simulink model "bit_simulink"  (R2023b)
settings: Solver=FixedStepAuto  StartTime=0.0  StopTime=1000  FixedStep=0.001  MaxStep=0.005  RelTol=1e-3
values from neighbouring files (symbols this model uses):
  d_theta_dt_0 = [0.,0.,0.,0.,0.,0.,0.,0.,0.]'    [Initialization.m]    (also in init_func.m; init_func_env_test.m; main_func.m; sim_loop_rust.m = double([0.,0.,0.,0.,0.,0.,0.,0.,0.]'))
  theta_0 = [0.,0.4*pi/180.0,0.4*pi/180.0,0.1*pi/180.0,0.1*pi/180.0,0.1*pi/180.0,0.,0.1,40*pi/180]'    [Initialization.m]    (also in init_func.m = [0,0,0,0,0,0,0,0,0,0]'; init_func_env_test.m = [0,0,0,0,0,0,0,0,0,0]'; main_func.m = [0.,0.4*pi/180.0,0.4*pi/180.0,0.1*pi/180.0,0.1*pi/180.0,0.1*; sim_loop_rust.m = 0*[0,0,0,0,0,0.0,0,0,-40*pi/180]')
  x0 = [d_theta_dt_0; theta_0; hs_rw]    [main.m]    (also in main_func.m; opt_ql.m = ones(91,1); sim_loop_rust.m = x0*1.01; sim_loop_wind.m)
undefined symbols (not defined in the file or in its folder): Klqr, Klqr_p, Klqr_r, ns, p, Qcm, r_pit, r_roll, rstr, sstr
settings Model: Creator=bholder  LastModifiedBy=bholder

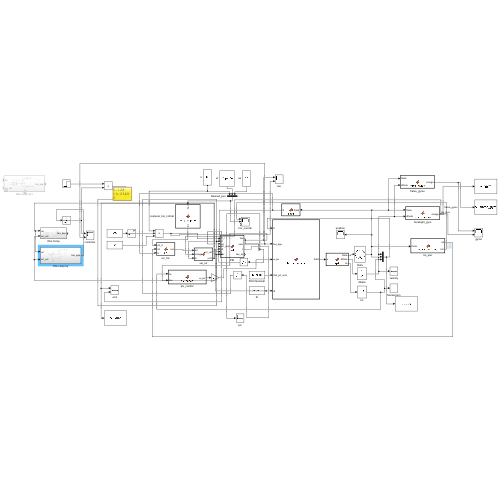
[thumbnail: Simulink's stored preview of the top-level diagram]
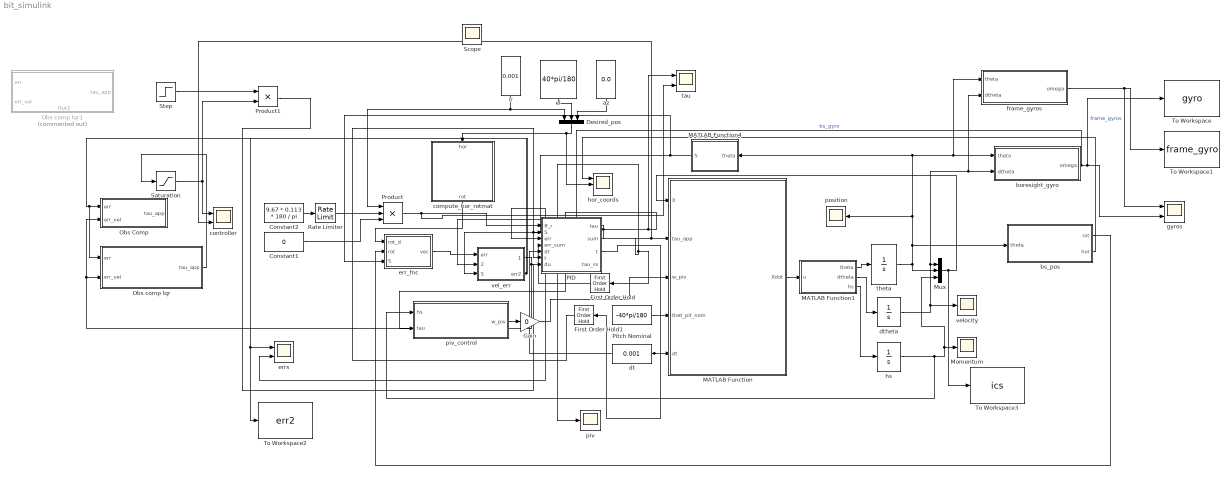
== system bit_simulink ==
  Constant1 : Constant  Value=0
  Constant2 : Constant  Value=9.67 * 0.113 * 180 / pi
  Desired_pos : Mux  Inputs=3
  First Order Hold : FirstOrderHold  InitialOutput=zeros(3,1)  ErrorTolerance=10  AllowContinuousInput=on
  First Order Hold1 : FirstOrderHold  ErrorTolerance=10  AllowContinuousInput=on
  Gain : Gain  Gain=0
  MATLAB Function : MATLAB Function  TreatAsAtomicUnit=on
  MATLAB Function1 : MATLAB Function  TreatAsAtomicUnit=on
  MATLAB Function4 : MATLAB Function  TreatAsAtomicUnit=on
  Momentum : Scope
  Mux : Mux  Inputs=3
  Obs Comp : Subsystem
  Obs comp lqr : Subsystem
  Obs comp lqr1 : Subsystem  Commented=on
      settings: PortSchema="{\"entries\":[{\"content\":{\"sides\":[{\"content\":{\"connectorIds\":[\"In1\",\"In2\"]},\"type\":\"ConnectorPlacement.EquallySpacedRectSide\",\"uuid\":\"f9d8c282-cd97-41f4-aac3-c7cf1abd67fe\"},{\"content\":{\"connectorIds\":[\"Out1\"],\"side\":\"RIGHT\"},\"type\":\"ConnectorPlacement.EquallySpacedRectSide\",\"uuid\":\"09112819-b147-4feb-a738-ff15dc4c45ff\"},{\"content\":{\"side\":\"TOP\"},\"type\":\"ConnectorPlacement.EquallySpacedRectSide\",\"uuid\":\"cd0336e0-d679-46ce-94e8-540b25d3be2c\"},{\"content\":{\"connectorIds\":[\"Out2\"],\"side\":\"BOTTOM\"},\"type\":\"ConnectorPlacement.EquallySpacedRectSide\",\"uuid\":\"8134ff57-d3b4-4301-9a67-166d46c0ba79\"}]},\"type\":\"ConnectorPlacement.EquallySpacedConnector\",\"uuid\":\"7e617e88-15c2-4d81-bfcb-fc8957304092\"}],\"packageUris\":[\"http://schema.mathworks.com/mf0/Connector/R2020b\"],\"version\":\"1.0\"}"
  PID : MATLAB Function  TreatAsAtomicUnit=on
  Pitch Nominal : Constant  Value=-40*pi/180
  Product : Product  Inputs=3
  Product1 : Product
  Rate Limiter : RateLimiter  RisingSlewLimit=15  FallingSlewLimit=-0.25  SampleTimeMode=inherited
  Saturation : Saturate  UpperLimit=1  LowerLimit=-1
  Step : Step  Time=0  Before=1  SampleTime=0
  To Workspace : ToWorkspace  VariableName=gyro  SaveFormat=Timeseries  SampleTime=-1
  To Workspace1 : ToWorkspace  VariableName=frame_gyro  SaveFormat=Timeseries  SampleTime=-1
  To Workspace2 : ToWorkspace  VariableName=err2  SaveFormat=Timeseries  SampleTime=-1
  To Workspace3 : ToWorkspace  VariableName=ics  SaveFormat=Timeseries  SampleTime=-1
      settings: MaxDataPoints=1
  az : Constant  Value=0.0
  boresight_gyro : MATLAB Function  TreatAsAtomicUnit=on
  bs_pos : MATLAB Function  TreatAsAtomicUnit=on
  compute_hor_rotmat : MATLAB Function  TreatAsAtomicUnit=on
  controller : Scope  NumInputPorts=2
  dt : Constant  Value=0.001
  dtheta : Integrator  InitialCondition=d_theta_dt_0  ContinuousStateAttributes='dtheta'
  el : Constant  Value=40*pi/180
  err_fnc : MATLAB Function  TreatAsAtomicUnit=on
  errs : Scope  NumInputPorts=2
  frame_gyros : MATLAB Function  TreatAsAtomicUnit=on
  gyros : Scope  NumInputPorts=2
  hor_coords : Scope  NumInputPorts=3
  hs : Integrator  InitialCondition=x0(19:21)  LimitOutput=on  UpperSaturationLimit=4*pi*4.5  LowerSaturationLimit=-4*pi*4.5  ContinuousStateAttributes='hs'
  ir : Constant  Value=0.001
  piv : Scope
  piv_control : MATLAB Function  TreatAsAtomicUnit=on
  position : Scope
  tau : Scope  NumInputPorts=2
  theta : Integrator  InitialCondition=theta_0  UpperSaturationLimit=1  LowerSaturationLimit=0  WrapState=on  ContinuousStateAttributes='theta'
  vel_err : MATLAB Function  TreatAsAtomicUnit=on
  velocity : Scope
  Scope : Scope
  wires:
  MATLAB Function/1(Xdot) -> MATLAB Function1/1(u)
  MATLAB Function1/2(dtheta) -> dtheta/1
  MATLAB Function1/1(theta) -> theta/1
  theta/1 -> Mux/2, bs_pos/1(theta), MATLAB Function4/1(theta), frame_gyros/1(theta), boresight_gyro/1(theta), position/1
  dtheta/1 -> frame_gyros/2(dtheta), boresight_gyro/2(dtheta), Mux/1, velocity/1
  Mux/1 -> MATLAB Function/1(X), To Workspace3/1
  Pitch Nominal/1 -> MATLAB Function/4(thet_pit_nom)
  dt/1 -> MATLAB Function/5(dt), PID/5(dt)
  MATLAB Function1/3(hs) -> hs/1
  hs/1 -> piv_control/1(hs), Momentum/1, Mux/3
  ir/1 -> Product/1, Desired_pos/1
  Desired_pos/1 -> compute_hor_rotmat/1(hor), hor_coords/2
  az/1 -> Desired_pos/3
  el/1 -> Desired_pos/2
  compute_hor_rotmat/1(rot) -> err_fnc/1(rot_d)
  bs_pos/1(rot) -> err_fnc/2(rot)
  err_fnc/1(vec) -> vel_err/1(err)
  MATLAB Function4/1(S) -> err_fnc/3(S), vel_err/3(S), PID/2(S)
  PID/2(sum) -> piv/1, First Order Hold/1
  First Order Hold/1 -> PID/4(err_sum)
  Constant2/1 -> Rate Limiter/1
  PID/1(tau) -> controller/2, MATLAB Function/2(tau_app), piv_control/2(tau), tau/1
  Rate Limiter/1 -> Product/2
  Constant1/1 -> Product/3
  Product/1 -> tau/2, PID/1(ff_r)
  piv_control/1(w_piv) -> Gain/1
  Gain/1 -> MATLAB Function/3(w_piv)
  PID/3(t) -> First Order Hold1/1
  First Order Hold1/1 -> PID/6("t ")
  boresight_gyro/1(omega) -> To Workspace/1, gyros/2, vel_err/2(omega)  "bs_gyro"
  bs_pos/2(hor) -> hor_coords/1
  frame_gyros/1(omega) -> gyros/1, To Workspace1/1  "frame_gyros"
  vel_err/1(err_vel) -> Obs Comp/2(err_vel), Obs comp lqr/2(err_vel), PID/3(err), errs/2
  vel_err/2(err2) -> To Workspace2/1, errs/1, Obs comp lqr/1(err), Obs Comp/1(err)
  Saturation/1 -> controller/1, Product1/2
  Product1/1 -> PID/7(du)
  Step/1 -> Product1/1
  Obs comp lqr/1(tau_app) -> Saturation/1

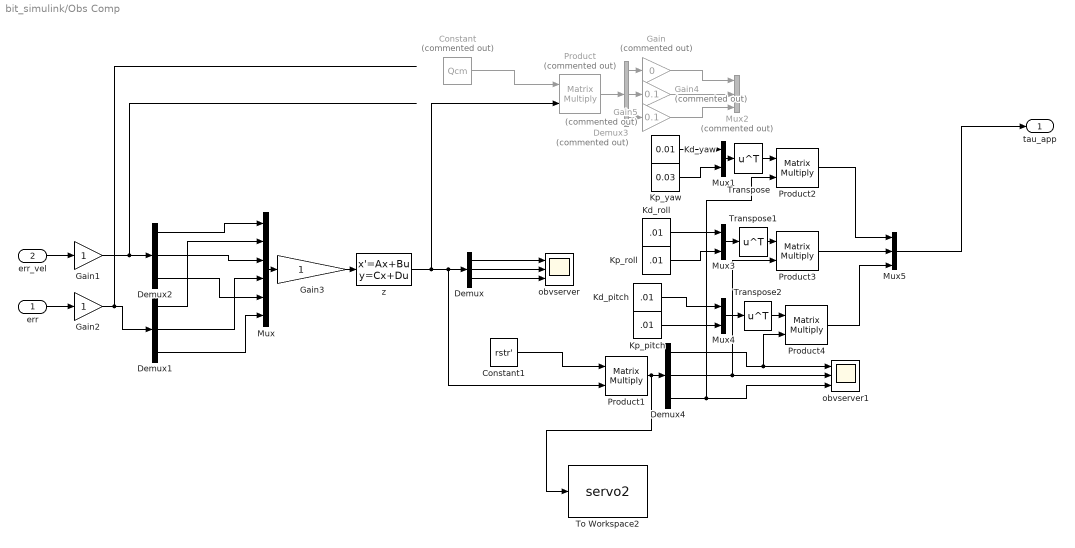
== system bit_simulink/Obs Comp ==
  err : Inport
  err_vel : Inport  Port=2
  Constant : Constant  Commented=on  Value=Qcm
  Constant1 : Constant  Value=rstr'
  Demux{,1..2,4} (4 alike) : Demux  Outputs=3
  Demux3 : Demux  Commented=on  Outputs=3
  Gain : Gain  Commented=on  Gain=0
  Gain1 : Gain
  Gain2 : Gain
  Gain3 : Gain
  Gain4 : Gain  Commented=on  Gain=0.1
  Gain5 : Gain  Commented=on  Gain=0.1
  Kd_pitch : Constant  Value=.01
  Kd_roll : Constant  Value=.01
  Kd_yaw : Constant  Value=0.01
  Kp_pitch : Constant  Value=.01
  Kp_roll : Constant  Value=.01
  Kp_yaw : Constant  Value=0.03  VectorParams1D=off
  Mux : Mux  Inputs=6
  Mux1 : Mux  Inputs=2
  Mux2 : Mux  Commented=on  Inputs=3
  Mux3 : Mux  Inputs=2
  Mux4 : Mux  Inputs=2
  Mux5 : Mux  Inputs=3
  Product : Product  Commented=on  Multiplication=Matrix(*)
  Product{1..4} (4 alike) : Product  Multiplication=Matrix(*)
  To Workspace2 : ToWorkspace  VariableName=servo2  SaveFormat=Timeseries  SampleTime=-1
  Transpose : Math  Operator=transpose
  Transpose1 : Math  Operator=transpose
  Transpose2 : Math  Operator=transpose
  obvserver : Scope  NumInputPorts=3
  obvserver1 : Scope  NumInputPorts=3
  z : StateSpace  A=sstr  B=rstr  C=eye(ns*3)  D=zeros(ns*3,6)  InitialCondition=0
  tau_app : Outport
  wires:
  Demux/1 -> obvserver/1
  Demux1/1 -> Mux/2
  Demux2/1 -> Mux/1
  Demux2/2 -> Mux/3
  Demux2/3 -> Mux/5
  Demux1/2 -> Mux/4
  Demux1/3 -> Mux/6
  Mux/1 -> Gain3/1
  z/1 -> Product/2, Product1/2, Demux/1
  Demux/2 -> obvserver/2
  Demux/3 -> obvserver/3
  Constant/1 -> Product/1
  Product/1 -> Demux3/1
  Demux3/1 -> Gain/1
  Gain/1 -> Mux2/1
  err_vel/1 -> Gain1/1
  err/1 -> Gain2/1
  Gain1/1 -> Demux2/1
  Gain2/1 -> Demux1/1
  Constant1/1 -> Product1/1
  Product1/1 -> To Workspace2/1, Demux4/1
  Demux4/1 -> Product4/2, obvserver1/1
  Demux4/2 -> Product3/2, obvserver1/2
  Demux4/3 -> Product2/2, obvserver1/3
  Gain3/1 -> z/1
  Kd_yaw/1 -> Mux1/1
  Kp_yaw/1 -> Mux1/2
  Kd_roll/1 -> Mux3/1
  Kp_roll/1 -> Mux3/2
  Kd_pitch/1 -> Mux4/1
  Kp_pitch/1 -> Mux4/2
  Mux1/1 -> Transpose/1
  Transpose/1 -> Product2/1
  Mux3/1 -> Transpose1/1
  Transpose1/1 -> Product3/1
  Mux4/1 -> Transpose2/1
  Transpose2/1 -> Product4/1
  Demux3/2 -> Gain4/1
  Demux3/3 -> Gain5/1
  Gain5/1 -> Mux2/3
  Gain4/1 -> Mux2/2
  Product2/1 -> Mux5/1
  Product3/1 -> Mux5/2
  Product4/1 -> Mux5/3
  Mux5/1 -> tau_app/1

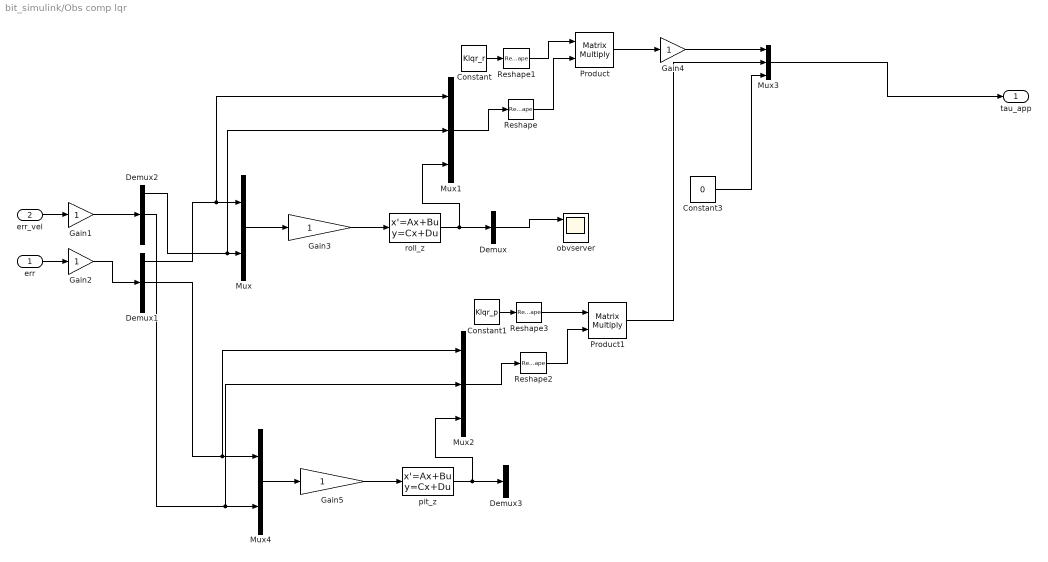
== system bit_simulink/Obs comp lqr ==
  err : Inport
  err_vel : Inport  Port=2
  Constant : Constant  Value=Klqr_r
  Constant1 : Constant  Value=Klqr_p
  Constant3 : Constant  Value=0
  Demux : Demux  Outputs=1
  Demux1 : Demux  Outputs=3
  Demux2 : Demux  Outputs=3
  Demux3 : Demux  Outputs=1
  Gain{1..5} (5 alike) : Gain
  Mux : Mux  Inputs=2
  Mux1 : Mux  Inputs=3
  Mux2 : Mux  Inputs=3
  Mux3 : Mux  Inputs=3
  Mux4 : Mux  Inputs=2
  Product : Product  Multiplication=Matrix(*)
  Product1 : Product  Multiplication=Matrix(*)
  Reshape : Reshape  OutputDimensionality=Column vector (2-D)
  Reshape1 : Reshape  OutputDimensionality=Row vector (2-D)
  Reshape2 : Reshape  OutputDimensionality=Column vector (2-D)
  Reshape3 : Reshape  OutputDimensionality=Row vector (2-D)
  obvserver : Scope  NumInputPorts=3
  pit_z : StateSpace  A=p  B=r_pit  C=eye(ns)  D=zeros(ns,2)  InitialCondition=zeros(ns,1)
  roll_z : StateSpace  A=p  B=r_roll  C=eye(ns)  D=zeros(ns,2)  InitialCondition=zeros(ns,1)
  tau_app : Outport
  wires:
  Demux/1 -> obvserver/1
  Demux2/1 -> Mux1/2, Mux/2
  Mux/1 -> Gain3/1
  roll_z/1 -> Mux1/3, Demux/1
  Constant/1 -> Reshape1/1
  Product/1 -> Gain4/1
  err_vel/1 -> Gain1/1
  err/1 -> Gain2/1
  Gain1/1 -> Demux2/1
  Gain2/1 -> Demux1/1
  Gain3/1 -> roll_z/1
  Gain4/1 -> Mux3/1
  Mux3/1 -> tau_app/1
  Demux1/1 -> Mux1/1, Mux/1
  Constant3/1 -> Mux3/3
  Mux1/1 -> Reshape/1
  Reshape/1 -> Product/2
  Reshape1/1 -> Product/1
  Mux2/1 -> Reshape2/1
  Product1/1 -> Mux3/2
  Reshape3/1 -> Product1/1
  Gain5/1 -> pit_z/1
  Constant1/1 -> Reshape3/1
  pit_z/1 -> Mux2/3, Demux3/1
  Reshape2/1 -> Product1/2
  Demux1/2 -> Mux2/1, Mux4/1
  Demux2/2 -> Mux2/2, Mux4/2
  Mux4/1 -> Gain5/1

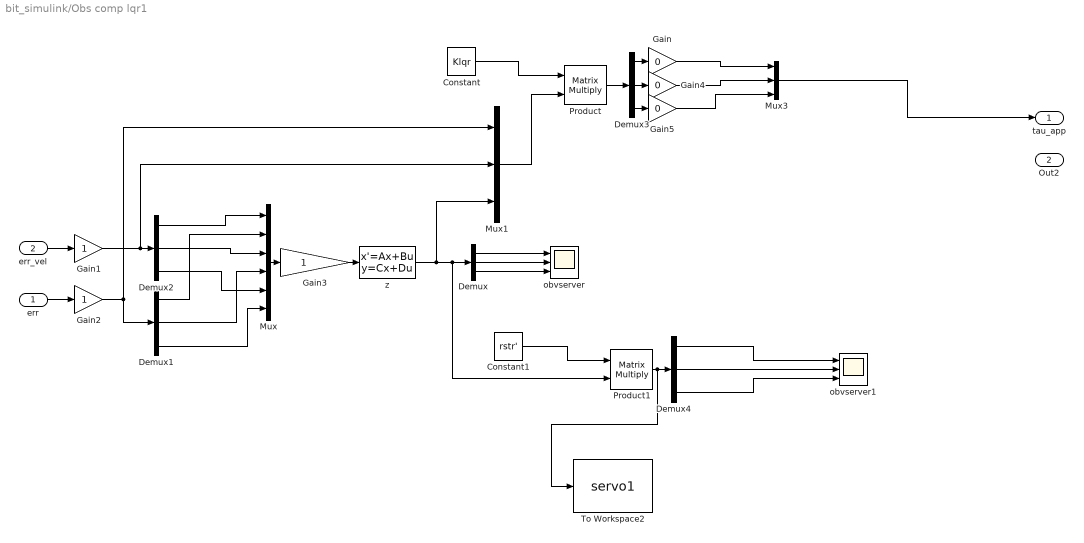
== system bit_simulink/Obs comp lqr1 ==
  err : Inport
  err_vel : Inport  Port=2
  Constant : Constant  Value=Klqr
  Constant1 : Constant  Value=rstr'
  Demux{,1..4} (5 alike) : Demux  Outputs=3
  Gain : Gain  Gain=0
  Gain1 : Gain
  Gain2 : Gain
  Gain3 : Gain
  Gain4 : Gain  Gain=0
  Gain5 : Gain  Gain=0
  Mux : Mux  Inputs=6
  Mux1 : Mux  Inputs=3
  Mux3 : Mux  Inputs=3
  Product : Product  Multiplication=Matrix(*)
  Product1 : Product  Multiplication=Matrix(*)
  To Workspace2 : ToWorkspace  VariableName=servo1  SaveFormat=Timeseries  SampleTime=-1
  obvserver : Scope  NumInputPorts=3
  obvserver1 : Scope  NumInputPorts=3
  z : StateSpace  A=sstr  B=rstr  C=eye(ns*3)  D=zeros(ns*3,6)  InitialCondition=0
  tau_app : Outport
  Out2 : Outport  Port=2
  wires:
  Demux/1 -> obvserver/1
  Demux1/1 -> Mux/2
  Demux2/1 -> Mux/1
  Demux2/2 -> Mux/3
  Demux2/3 -> Mux/5
  Demux1/2 -> Mux/4
  Demux1/3 -> Mux/6
  Mux/1 -> Gain3/1
  z/1 -> Mux1/3, Product1/2, Demux/1
  Demux/2 -> obvserver/2
  Demux/3 -> obvserver/3
  Constant/1 -> Product/1
  Product/1 -> Demux3/1
  Demux3/1 -> Gain/1
  Gain/1 -> Mux3/1
  err_vel/1 -> Gain1/1
  err/1 -> Gain2/1
  Gain1/1 -> Mux1/2, Demux2/1
  Gain2/1 -> Demux1/1, Mux1/1
  Constant1/1 -> Product1/1
  Product1/1 -> To Workspace2/1, Demux4/1
  Demux4/1 -> obvserver1/1
  Demux4/2 -> obvserver1/2
  Demux4/3 -> obvserver1/3
  Gain3/1 -> z/1
  Demux3/2 -> Gain4/1
  Demux3/3 -> Gain5/1
  Mux1/1 -> Product/2
  Gain5/1 -> Mux3/3
  Gain4/1 -> Mux3/2
  Mux3/1 -> tau_app/1

== matlab function bit_simulink/vel_err ==
  data: err input; err_vel output; omega input; S input; err2 output
function [err_vel, err2] = fcn(err, omega, S)

    d_thet = inv(S) * omega;

    dr = d_thet(1);
    dp = d_thet(2);
    dy = d_thet(3);


    err2 = S'*S*err;
    % err2 = err;

    er  = err2(1);
    ep = err2(2);
    ey = err2(3);

    %% yaw

    max_v = .01;
    slope = 2;
    yd = 1*max_v * erf(slope*ey);

    %% pitch
    max_v = 0.0025;
    slope = 10*.025;
    pd = 1*max_v  * erf(slope*ep);

    %% roll

    max_v = 0.00025;
    slope = 0.25*150;
    rd = 1*max_v * erf(slope*er);
    
    err_vel = [rd-dr;
               pd-dp;
               yd-dy];

== matlab function bit_simulink/frame_gyros ==
  data: theta input; omega output; dtheta input
function omega  = frame_gyros(theta,dtheta)
%UNTITLED2 Summary of this function goes here
%   Detailed explanation goes here
z_n = [0.0, 1.0, 0.0, 1.0, 0.0, 0.0, 0.0, 1.0, 0.0;
       0.0, 0.0, 1.0, 0.0, 1.0, 0.0, 0.0, 0.0, 1.0;
       1.0, 0.0, 0.0, 0.0, 0.0, 1.0, 1.0, 0.0, 0.0];

s7 = zeros(3,7);
s8 = zeros(3,8);

s9 = zeros(3,9);
for i = 1:9
    Cn = axis2rot(z_n(:,i), theta(i));
    s9(:,i) = z_n(:,i);
    s9 = Cn*s9; 

    if i == 7
        s7 = s9(:,1:7);
    elseif i == 8
        s8 = s9(:,1:8);
    end
end

om_yaw = s7 * dtheta(1:7);
om_roll = s8 * dtheta(1:8);

om_pit = s9 * dtheta;
omega = zeros(3,1);

omega = [om_roll(1); om_pit(2); om_yaw(3)];

end

== matlab function bit_simulink/MATLAB Function1 ==
  data: u input; theta output; dtheta output; hs output
function [theta, dtheta, hs] = split(u)
    
    dtheta = u(1:9);
    theta = u(10:18);
    hs = u(19:21);
end

== matlab function bit_simulink/MATLAB Function ==
  data: X input; Xdot output; tau_app input; w_piv input; thet_pit_nom input; dt input
function Xdot  = bit_propagator(X, tau_app, w_piv, thet_pit_nom, dt)
    
    piv_flag = true;
    tau_max_piv = 5;

    [ndof, g0, r_n1_n, z_n, p_n, m_n, c_n, ...
    i_n, m_w_n,  i_rw, bear_k_cst, bear_c_cst, k_d, b_d, ...
    w_rw_max, w_rw_nom, hs_rw, hs_rw_max, a_flex, b_flex, a_df, b_df] = init_func();

    %split the state

    theta = X(10:18);
    dtheta = X(1:9);
    hs = X(19:21);

    tau_applied = zeros(9,1);
    tau_applied(7:9) = tau_app;
    
    %extract RW torque.
    tau_rw = tau_applied(7);
    tau_applied(7) = 0;  


    dw_piv = 0;
    % set pivot speed in dtheta...
    if piv_flag == true
        dtheta(6) = w_piv;
        dw_ppiv = (w_piv - dtheta(6))/dt;
    end
    
    %%
    Pot = compute_potential_energy_term(theta, c_n, z_n, m_n, r_n1_n, g0);

    theta_spring = theta;
    theta_spring(9) = theta(9) - thet_pit_nom;
    
    spring = k_d.*theta_spring;
    damp = b_d.*dtheta;
    
    %place holder
    [R,r, d_hs] = RW_terms(theta, dtheta, z_n, hs, tau_rw, hs_rw_max);
       
    %calculate joint torques from gravity elasticity and damnping according
    %to eq 3.37
    torques = tau_applied - (Pot + spring + damp + R + r);
 
    % M = compute_mass_matrix(theta, z_n, r_n1_n, m_w_n, p_n);

    % M = mass_mat_func(theta);
    M = mass_mat_func_gb(theta);

    M_decomp = chol(M);

    ddtheta = M_decomp\((M_decomp')\torques);

    unlock = [1;1;1;1;1;1;1;1;1];

    ddtheta = ddtheta.*unlock;

    if piv_flag == true
        prop_err = 10;
        int_err = 0;
        kp = 1;
        ki = 0.5;
        prop_err = dw_piv - ddtheta(6);
        int_err = int_err + prop_err;
        tau_piv = torques(6);

        while abs(prop_err) > 1e-9
            
            tau_piv = tau_piv + ((kp*prop_err) + (ki*int_err));
            if abs(tau_piv) > tau_max_piv
                tau_piv = sign(tau_piv) * tau_max_piv;
                torques(6) = tau_piv;

                ddtheta = M_decomp\((M_decomp')\torques);
                break
            end
            torques(6) = tau_piv;

            ddtheta = M_decomp\((M_decomp')\torques);
            prop_err = dw_piv - ddtheta(6);
            int_err = int_err + prop_err;
        end
    end

    tau_gond = M(7:9,7:9) * ddtheta(7:9);
    % tau_gond(1) = tau_rw

    Xdot = [ddtheta; dtheta; d_hs];
    
end

== matlab function bit_simulink/boresight_gyro ==
  data: theta input; omega output; dtheta input
function omega  = comp_ang_vel(theta,dtheta)
%UNTITLED2 Summary of this function goes here
%   Detailed explanation goes here
z_n = [0.0, 1.0, 0.0, 1.0, 0.0, 0.0, 0.0, 1.0, 0.0;
       0.0, 0.0, 1.0, 0.0, 1.0, 0.0, 0.0, 0.0, 1.0;
       1.0, 0.0, 0.0, 0.0, 0.0, 1.0, 1.0, 0.0, 0.0];

s9 = zeros(3,9);
for i = 1:9
    Cn = axis2rot(z_n(:,i), theta(i));
    s9(:,i) = z_n(:,i);
    s9 = Cn*s9;    
end

omega = s9 * dtheta;

end

== matlab function bit_simulink/bs_pos ==
  data: theta input; rot output; hor output
function [rot, hor]  = comp_ang_pos(theta)
%UNTITLED2 Summary of this function goes here
%   Detailed explanation goes here
    z_n = [0.0, 1.0, 0.0, 1.0, 0.0, 0.0, 0.0, 1.0, 0.0;
           0.0, 0.0, 1.0, 0.0, 1.0, 0.0, 0.0, 0.0, 1.0;
           1.0, 0.0, 0.0, 0.0, 0.0, 1.0, 1.0, 0.0, 0.0];
    
    C = (eye(3));
    for i = 1:9
        C = axis2rot(z_n(:,i), theta(i)) * C;
    end
    rot = C;
    
    el = asin(C(1,3)); %roll
    ir = atan2(C(2,3), C(3,3)); %pitch 
    az = atan2(-C(1,2), C(1,1)); %yaw

    hor = [ir;el;az];

end

== matlab function bit_simulink/compute_hor_rotmat ==
  data: hor input; rot output
function rot  = comp_ang_rot(hor)
    %UNTITLED2 Summary of this function goes here
    %   Detailed explanation goes here
    z_n = [ 1.0, 0.0, 0.0;
            0.0, 1.0, 0.0;
            0.0, 0.0, 1.0];
    ir = hor(1);
    el = hor(2);
    az = hor(3);
    
    
    rot = axis2rot(z_n(:,1), ir) * axis2rot(z_n(:,2), -el) * axis2rot(z_n(:,3), -az);

end

== matlab function bit_simulink/err_fnc ==
  data: rot_d input; vec output; rot input; S input
function vec = err(rot_d, rot, S)

    rot_e = rot_d * rot';
    
    % yaw_err = atan2(eq_err_rot(2,3), eq_err_rot(3,3));
    % pit_err = asin(-eq_err_rot(1,3));
    % roll_err = atan2(eq_err_rot(1,2), eq_err_rot(1,1));

    roll_e = atan2(rot_e(2,3), rot_e(3,3));
    pitch_e = asin(-rot_e(1,3));
    xpitch_e = atan2(rot_e(1,2), rot_e(1,1));

    vec= inv(S) * [roll_e; pitch_e; xpitch_e];
    % vec= [roll_err; pit_err; yaw_err];
end

== matlab function bit_simulink/PID ==
  data: ff_r input; S input; tau output; err input; err_sum input; sum output; dt input; t input; t output; tau_ss output; du input
function [tau, sum, t, tau_ss] = pid(ff_r, S, err, err_sum, dt, t, du)

    mapped_err = err;
    sum = err_sum*0.99995;

    t = t + dt;


    % if norm(err) < 0.001 && t > 4
        sum = sum + mapped_err*dt;
    % end

    kp = 1*diag([50, 200, 50])/1;
    ki = diag([200, 200, 400])/2;

    % v1 = dist_u(1:4);
    % v2 = dist_u(5:8);
    % v3 = dist_u(9:12);
    % 
    % ky = .1*[-1, -1, -1, -1];
    % kr = .1*[-1, -.1, -1, -.1];
    % kpi = 0.075*[-1, -1, -1, -1];
    % 
    % du = [kr*v1; kpi*v2; ky*v3];
    % sv_u = [du(2); du(3); du(1)];

    pid = (kp * mapped_err + ki * sum) + du;

    tau = zeros(3,1);

    tau(1) = -pid(3);
    tau(2) = pid(1) + ff_r;
    tau(3) = pid(2);

    tau_ss = zeros(3,1);

    tau_ss(1) = -pid(3);
    tau_ss(2) = pid(1);
    tau_ss(3) = pid(2);

end

== matlab function bit_simulink/MATLAB Function4 ==
  data: theta input; S output
function S = gmm(theta)

    roll = theta(8);
    pitch = theta(9);

    S = [cos(pitch), 0, -cos(roll)*sin(pitch);
        0, 1, sin(roll);
        sin(pitch), 0, cos(pitch)*cos(roll)];

== matlab function bit_simulink/piv_control ==
  data: hs input; w_piv output; tau input
function w_piv = piv_speed(hs, tau)

    

    rw_tau = tau(1);
    gain1 = 2.25e-6;
    k_flight_train= 0.001745329251994;
    i_rw= 2*4.5;
    rw_w = hs(3) / i_rw;
    gain2= 0.001 * (4.5e-7 * (sqrt(gain1 / (i_rw * k_flight_train))));
    
    w_piv = gain1 * (pi - rw_w) + gain2 * rw_tau;
end
